simulink model "UFFR"  (Simulink 8.3)
settings: Solver=ode45  StartTime=0.0  StopTime=10  RelTol=1e-3
settings Model: Creator=Administrator  LastModifiedBy=JimmyChen
settings DataIOCC: SignalLoggingSaveFormat=Dataset
settings DebuggingCC: UnderspecifiedInitializationDetection=Simplified  StateNameClashWarn=none
settings GRTTargetCC: CombineOutputUpdateFcns=on  GRTInterface=off

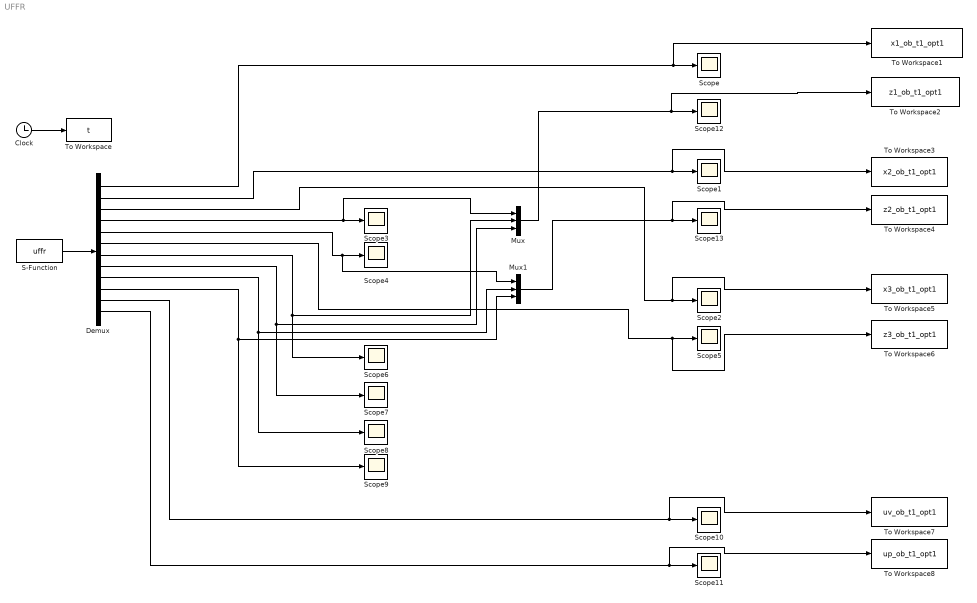
== system UFFR ==
  Clock : Clock
  Demux : Demux  Outputs=12
  Mux : Mux  Inputs=3
  Mux1 : Mux  Inputs=3
  S-Function : S-Function  FunctionName=uffr  EnableBusSupport=off
  Scope{,1..13} (14 alike) : Scope
      Scope10 settings: SaveName=ScopeData10
      Scope11 settings: SaveName=ScopeData11
      Scope12 settings: SaveName=ScopeData12
      Scope13 settings: SaveName=ScopeData13
      Scope2 settings: SaveName=ScopeData2
      Scope3 settings: SaveName=ScopeData3
      Scope4 settings: SaveName=ScopeData4
      Scope5 settings: SaveName=ScopeData5
      Scope6 settings: SaveName=ScopeData6
      Scope7 settings: SaveName=ScopeData7
      Scope8 settings: SaveName=ScopeData8
      Scope9 settings: SaveName=ScopeData9
  To Workspace : ToWorkspace  VariableName=t  SaveFormat=Timeseries  SampleTime=-1
  To Workspace1 : ToWorkspace  VariableName=x1_ob_t1_opt1  SaveFormat=Timeseries  SampleTime=-1
  To Workspace2 : ToWorkspace  VariableName=z1_ob_t1_opt1  SaveFormat=Timeseries  SampleTime=-1
  To Workspace3 : ToWorkspace  VariableName=x2_ob_t1_opt1  SaveFormat=Timeseries  SampleTime=-1
  To Workspace4 : ToWorkspace  VariableName=z2_ob_t1_opt1  SaveFormat=Timeseries  SampleTime=-1
  To Workspace5 : ToWorkspace  VariableName=x3_ob_t1_opt1  SaveFormat=Timeseries  SampleTime=-1
  To Workspace6 : ToWorkspace  VariableName=z3_ob_t1_opt1  SaveFormat=Timeseries  SampleTime=-1
  To Workspace7 : ToWorkspace  VariableName=uv_ob_t1_opt1  SaveFormat=Timeseries  SampleTime=-1
  To Workspace8 : ToWorkspace  VariableName=up_ob_t1_opt1  SaveFormat=Timeseries  SampleTime=-1
  wires:
  S-Function/1 -> Demux/1
  Clock/1 -> To Workspace/1
  Demux/1 -> To Workspace1/1, Scope/1
  Demux/6 -> To Workspace6/1, Scope5/1
  Demux/7 -> Scope6/1, Mux/2
  Demux/8 -> Scope7/1, Mux/3
  Demux/9 -> Scope8/1, Mux1/2
  Demux/10 -> Scope9/1, Mux1/3
  Demux/11 -> To Workspace7/1, Scope10/1
  Demux/12 -> To Workspace8/1, Scope11/1
  Demux/4 -> Scope3/1, Mux/1
  Demux/5 -> Mux1/1, Scope4/1
  Mux/1 -> To Workspace2/1, Scope12/1
  Demux/2 -> To Workspace3/1, Scope1/1
  Mux1/1 -> To Workspace4/1, Scope13/1
  Demux/3 -> To Workspace5/1, Scope2/1
